simulink model "PCS"  (R2018b)
settings: Solver=FixedStepAuto  StartTime=0.0  StopTime=inf  RelTol=1e-3  EnableMultiTasking=on
libraries: embdlinuxlib x5, raspberrypilib x2, dspmtrx3 x1, visionanalysis x1, simulink x1, visiongeotforms x1
settings Model: SimulationMode=external  Creator=HP  LastModifiedBy=Double lee
settings SolverCC: PositivePriorityOrder=on  AutoInsertRateTranBlk=on
settings OptimizationCC: EnhancedBackFolding=on  PassReuseOutputArgsAs=Individual arguments  MaxStackSize=64  OptimizeBlockOrder=speed  DifferentSizesBufferReuse=on  OptimizationCustomize=off
settings DebuggingCC: ParameterTunabilityLossMsg=error
settings HardwareCC: ProdBitPerPointer=32  ProdBitPerSizeT=32  ProdBitPerPtrDiffT=32  ProdLargestAtomicInteger=Long  ProdLargestAtomicFloat=Double  ProdWordSize=32  ProdHWDeviceType=ARM Compatible->ARM Cortex
settings SFSimCC: MATLABDynamicMemAlloc=off
settings RTWCC: SystemTargetFile=ert.tlc  HardwareBoard=Raspberry Pi  TLCOptions="-aInlineSetEventsForThisBaseRateFcn=TLC_FALSE -aSuppressMultiTaskScheduler=TLC_FALSE  -aRateBasedStepFcn=0"  TemplateMakefile=ert_default_tmf  GenerateReport=on  Toolchain=GNU GCC Raspberry Pi  BuildConfiguration=Faster Runs  IncludeHyperlinkInReport=on  LaunchReport=on  GenerateTraceInfo=on  GenerateTraceReport=on  GenerateTraceReportSl=on  GenerateTraceReportSf=on  GenerateTraceReportEml=on
settings CodeAppCC: ForceParamTrailComments=on  IgnoreCustomStorageClasses=off  OperatorAnnotations=on  SimulinkDataObjDesc=on  SFDataObjDesc=on  InsertBlockDesc=on
settings ERTTargetCC: SupportContinuousTime=on  SupportVariableSizeSignals=on  ExtMode=on  ExtModeMexArgs='192.168.43.176' 0 17724

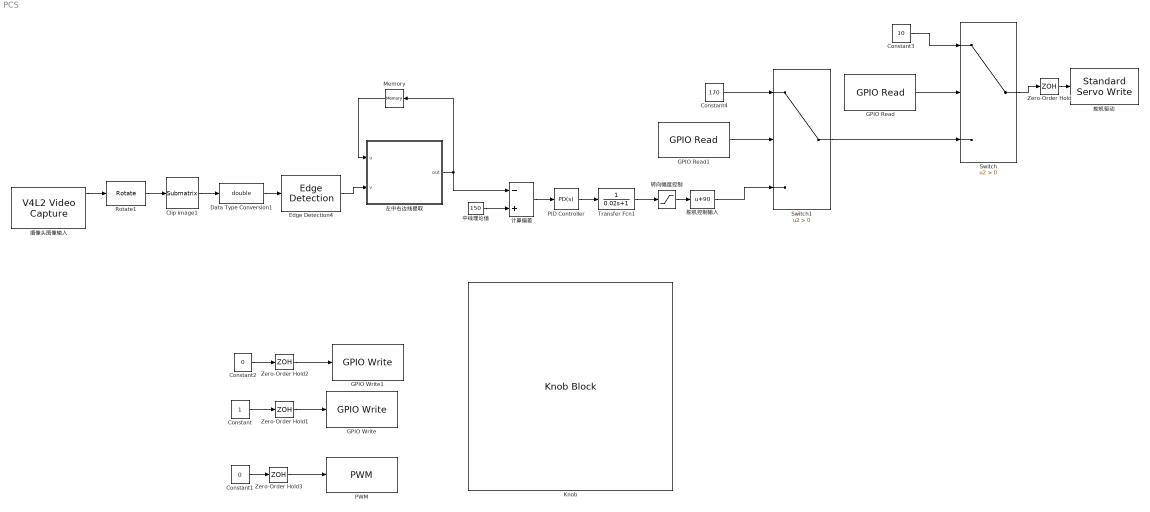
== system PCS ==
  Clip image1 : dspmtrx3/Submatrix  RowSpan=Range of rows  RowStartMode=Index  RowStartIndex=80  RowEndMode=Index  RowEndIndex=180  ColSpan=All columns  ColStartMode=First  ColStartIndex=1  ColEndMode=Last  ColEndIndex=1
  Constant : Constant
  Constant1 : Constant  Value=0
  Constant2 : Constant  Value=0
  Constant3 : Constant  Value=10
  Constant4 : Constant  Value=170
  Data Type Conversion1 : DataTypeConversion  OutDataTypeStr=double
  Edge Detection4 : visionanalysis/Edge Detection  method=Sobel  outputType=Binary image  userDefinedThreshold=on  thresholdSource=Specify via dialog  threshold=20  thresholdTuning=1  edgeThinning=on  threshold_canny=[0.25 0.60]  autoPercent=90  sigma=1  roundingMode=Floor  overflowMode=off  prodOutputMode=Binary point scaling  prodOutputWordLength=32  prodOutputFracLength=8  prodOutputSlope=2^-8  accumSlope=2^-8  outputSlope=2^-4
      settings: SourceProductName=Computer Vision System Toolbox  SourceProductBaseCode=VP
  GPIO Read : embdlinuxlib/GPIO Read  board=Pi 3 Model B+  gpio=26  internalResistor=Off  sampleTime=inf  direction=Input  blockPlatform=Raspberry Pi
      settings: SourceProductName=Simulink Support Package for Raspberry Pi Hardware  SourceProductBaseCode=RASPPI
  GPIO Read1 : embdlinuxlib/GPIO Read  board=Pi 3 Model B+  gpio=27  internalResistor=Off  sampleTime=inf  direction=Input  blockPlatform=Raspberry Pi
      settings: SourceProductName=Simulink Support Package for Raspberry Pi Hardware  SourceProductBaseCode=RASPPI
  GPIO Write : embdlinuxlib/GPIO Write  board=Pi 3 Model B+  gpio=23  direction=Output  blockPlatform=Raspberry Pi
      settings: SourceProductName=Simulink Support Package for Raspberry Pi Hardware  SourceProductBaseCode=RASPPI
  GPIO Write1 : embdlinuxlib/GPIO Write  board=Pi 3 Model B+  gpio=22  direction=Output  blockPlatform=Raspberry Pi
      settings: SourceProductName=Simulink Support Package for Raspberry Pi Hardware  SourceProductBaseCode=RASPPI
  Knob : KnobBlock  WebBlockId=163  ScaleMax=0.14999999999999999
  Memory : Memory
  PID Controller : simulink/Continuous/PID Controller  Controller=PD  Form=Parallel  TimeDomain=Continuous-time  SampleTime=-1  IntegratorMethod=Forward Euler  FilterMethod=Forward Euler  ControllerParametersSource=internal  P=0.8  I=1  D=0.0005  UseFilter=on  N=3  TunerSelectOption=Transfer Function Based (PID Tuner App)  InitialConditionSource=internal  InitialConditionForIntegrator=0  InitialConditionForFilter=0  DifferentiatorICPrevScaledInput=0  ExternalReset=none  TrackingMode=off  Kt=1  LimitOutput=off  UpperSaturationLimit=inf  LowerSaturationLimit=-inf  LinearizeAsGain=on  AntiWindupMode=none  Kb=1  POutMin=[]  POutMax=[]  IOutMin=[]  IOutMax=[]  DOutMin=[]  DOutMax=[]  NOutMin=[]  NOutMax=[]  SumOutMin=[]  SumOutMax=[]  SaturationOutMin=[]  SaturationOutMax=[]  PParamMin=[]  PParamMax=[]  IParamMin=[]  IParamMax=[]  DParamMin=[]  DParamMax=[]  NParamMin=[]  NParamMax=[]  KbParamMin=[]  KbParamMax=[]  KtParamMin=[]  KtParamMax=[]  KbOutMin=[]  KbOutMax=[]  KtOutMin=[]  KtOutMax=[]  IntegratorOutMin=[]  IntegratorOutMax=[]  FilterOutMin=[]  FilterOutMax=[]  SumI1OutMin=[]  SumI1OutMax=[]  SumI2OutMin=[]  SumI2OutMax=[]  SumI3OutMin=[]  SumI3OutMax=[]  SumI4OutMin=[]  SumI4OutMax=[]  SumDOutMin=[]  SumDOutMax=[]  DifferentiatorOutMin=[]  DifferentiatorOutMax=[]  FilterDiffOutCoefMin=[]  FilterDiffOutCoefMax=[]  ReciprocalOutMin=[]  ReciprocalOutMax=[]  SumDenOutMin=[]  SumDenOutMax=[]  SumNumOutMin=[]  SumNumOutMax=[]  DivideOutMin=[]  DivideOutMax=[]  IntegratorContinuousStateAttributes=''  IntegratorStateMustResolveToSignalObject=off  IntegratorRTWStateStorageClass=Auto  FilterContinuousStateAttributes=''  FilterStateMustResolveToSignalObject=off  FilterRTWStateStorageClass=Auto  ParallelPVariant=InternalParameters  IdealPVariant=Disabled  IVariant=Disabled  DVariant=InternalParameters  IntegratorVariant=Disabled  SatVariant=Disabled  AWVariant=Disabled  PCopyVariant=Disabled  TRVariant=Disabled  FdbkBlocksVariant=Forward  IdealPFdbkVariant=Disabled  SatFdbkVariant=Disabled  DerivativeFilterVariant=ContFilter  NVariant=InternalParameters  NCopyVariant=Disabled  FilterICVariant=InternalICsFilter  IntegratorICVariant=Disabled  ExternalResetVariant=Disabled  TRSumVariant=Passthrough  SumFdbkVariant=Disabled  SumVariant=Sum_PD
  PWM : raspberrypilib/PWM  board=Pi 3 Model B  Pin_=18  Frequency=100  blockPlatform=Raspberry Pi
      settings: SourceProductName=Simulink Support Package for Raspberry Pi Hardware  SourceProductBaseCode=RASPPI
  Rotate1 : visiongeotforms/Rotate  outSizeR=Expanded to fit rotated input image  src_angle=Specify via dialog  unit_angle=Degrees  angle=-pi/2  maxAngle=pi  dispImage=Top-left corner  method=Table lookup  fillVal=0  interpMethod=Bilinear  prodOutputMode=Binary point scaling  prodOutputWordLength=32  prodOutputFracLength=10  roundingMode=Nearest  overflowMode=on
      settings: SourceProductName=Computer Vision System Toolbox  LockScale=on
  Switch : Switch  Criteria=u2 > Threshold
  Switch1 : Switch  Criteria=u2 > Threshold
  Transfer Fcn1 : TransferFcn  Denominator=[0.02 1]
  Zero-Order Hold{,1..3} (4 alike) : ZeroOrderHold  SampleTime=0.05
  中线理论值 : Constant  Value=150
  左中右边线提取 : MATLAB Function  TreatAsAtomicUnit=on
  摄像头图像输入 : embdlinuxlib/V4L2 Video Capture  m_devName='/dev/video0'  roi=[0, 0, 640, 480]  imSizeSelection=320x240  imSize=[640, 480]  pixelFormat=RGB  pixelOrder=Planar  sampleTime=1/50  simOutput=Colorbars  blockPlatform=Raspberry Pi
      settings: SourceProductName=Simulink Support Package for Raspberry Pi Hardware  SourceProductBaseCode=RASPPI
  舵机控制输入 : Bias  Bias=90
  舵机驱动 : raspberrypilib/Standard Servo Write  board=Pi 3 Model B  Pin_=17  MinPulseDuration=0.9e-3  MaxPulseDuration=2.1e-3  blockPlatform=Raspberry Pi
      settings: SourceProductName=Simulink Support Package for Raspberry Pi Hardware  SourceProductBaseCode=RASPPI
  计算偏差 : Sum  Inputs=-+
  转向幅度控制 : Saturate  UpperLimit=85  LowerLimit=-85
  wires:
  Data Type Conversion1/1 -> Edge Detection4/1
  Rotate1/1 -> Clip image1/1
  Clip image1/1 -> Data Type Conversion1/1
  中线理论值/1 -> 计算偏差/2
  摄像头图像输入/1 -> Rotate1/1
  Zero-Order Hold/1 -> 舵机驱动/1
  转向幅度控制/1 -> 舵机控制输入/1
  Transfer Fcn1/1 -> 转向幅度控制/1
  Edge Detection4/1 -> 左中右边线提取/2(v)
  左中右边线提取/1(out) -> 计算偏差/1, Memory/1
  计算偏差/1 -> PID Controller/1
  Memory/1 -> 左中右边线提取/1(u)
  Constant1/1 -> Zero-Order Hold3/1
  Zero-Order Hold3/1 -> PWM/1
  PID Controller/1 -> Transfer Fcn1/1
  Constant3/1 -> Switch/1
  Constant4/1 -> Switch1/1
  舵机控制输入/1 -> Switch1/3
  Switch1/1 -> Switch/3
  Switch/1 -> Zero-Order Hold/1
  Constant2/1 -> Zero-Order Hold2/1
  Constant/1 -> Zero-Order Hold1/1
  Zero-Order Hold1/1 -> GPIO Write/1
  Zero-Order Hold2/1 -> GPIO Write1/1
  GPIO Read1/1 -> Switch1/2
  GPIO Read/1 -> Switch/2

== matlab function PCS/左中右边线提取 ==
  data: u input; out output; v input
function out= fcn(u,v)
border=zeros(2,1);
[~,max]=size(v);
    for x_left=1:u
        if v(62,u-x_left)==1
           
           break
        end
        border(1,1)=u-x_left;
    end
    for x_right=1:max-u
        if v(62,u+x_right)==1
           break
        end
          border(2,1)=u+x_right;
    end
    if border(2,1)-border(1,1)>=220
         border(1,1)=border(2,1)-209;
    end
   put= border(1,1)+border(2,1);
   out =put/2;
end
